simulink model "DaoBaoTin_20151230_Cau1abc"  (R2018a)
settings: Solver=FixedStepAuto  StartTime=0.0  StopTime=100.0  FixedStep=0.1  RelTol=1e-3
values from neighbouring files (symbols this model uses):
  b = 0.1    [thongso_cau1.m]
  k = 0.1    [thongso_cau1.m]
  m = 1    [thongso_cau1.m]
settings Model: Creator=20151  LastModifiedBy=20151
settings DataIOCC: ReturnWorkspaceOutputs=on
settings DebuggingCC: UnconnectedInputMsg=none  UnconnectedOutputMsg=none  UnconnectedLineMsg=none  SFMachineParentedDataDiag=error
settings SFSimCC: SimUseLocalCustomCode=on
settings RTWCC: RTWUseLocalCustomCode=on

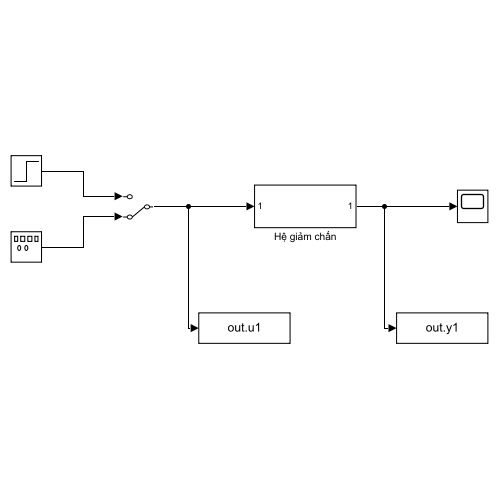
[thumbnail: Simulink's stored preview of the top-level diagram]
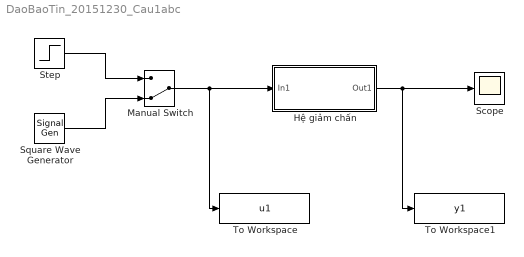
== system DaoBaoTin_20151230_Cau1abc ==
  Hệ giảm chấn : Subsystem
  Manual Switch : ManualSwitch  CurrentSetting=0
  Scope : Scope
  Square Wave Generator : SignalGenerator  WaveForm=random  Amplitude=20  Frequency=10  Units=rad/sec
  Step : Step  SampleTime=0.1
  To Workspace : ToWorkspace  VariableName=u1  SaveFormat=Timeseries  SampleTime=0.1
  To Workspace1 : ToWorkspace  VariableName=y1  SaveFormat=Timeseries  SampleTime=0.1
  wires:
  Step/1 -> Manual Switch/1
  Square Wave Generator/1 -> Manual Switch/2
  Hệ giảm chấn/1(Out1) -> To Workspace1/1, Scope/1
  Manual Switch/1 -> To Workspace/1, Hệ giảm chấn/1(In1)

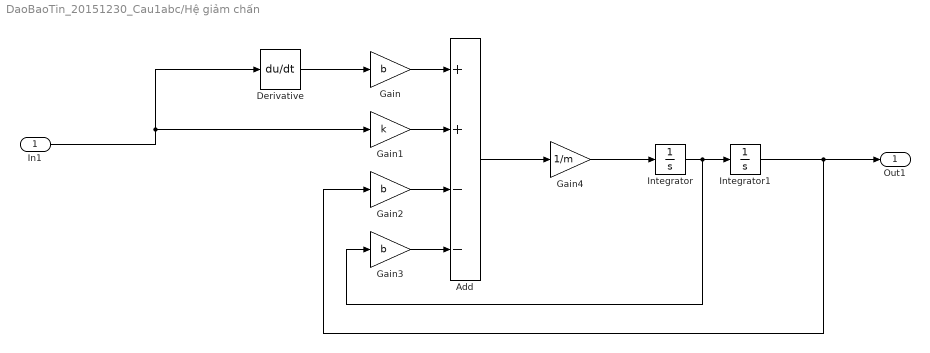
== system DaoBaoTin_20151230_Cau1abc/Hệ giảm chấn ==
  In1 : Inport
  Add : Sum  Inputs=++--
  Derivative : Derivative
  Gain : Gain  Gain=b
  Gain1 : Gain  Gain=k
  Gain2 : Gain  Gain=b
  Gain3 : Gain  Gain=b
  Gain4 : Gain  Gain=1/m
  Integrator : Integrator
  Integrator1 : Integrator
  Out1 : Outport
  wires:
  Gain/1 -> Add/1
  Gain1/1 -> Add/2
  Gain2/1 -> Add/3
  Gain3/1 -> Add/4
  Add/1 -> Gain4/1
  Derivative/1 -> Gain/1
  Gain4/1 -> Integrator/1
  Integrator/1 -> Gain3/1, Integrator1/1
  Integrator1/1 -> Gain2/1, Out1/1
  In1/1 -> Gain1/1, Derivative/1
